simulink model "SF048A_TqLoa"  (R2013b)
settings: Solver=FixedStepDiscrete  SolverMode=SingleTasking  StartTime=0.0  StopTime=1  FixedStep=0.002  RelTol=1e-3
values from neighbouring files (symbols this model uses):
  ARCHGLBPRM_2MILLISEC_SEC_F32 = DataDict.Constant    [SF048A_TqLoa_DataDict.m]
  ARCHGLBPRM_PIOVER180_ULS_F32 = DataDict.Constant    [SF048A_TqLoa_DataDict.m]
  GRVYTLCON_MTRPERSECSQD_F32 = DataDict.Constant    [SF048A_TqLoa_DataDict.m]
  HWAUTHYMIN_ULS_F32 = DataDict.Constant    [SF048A_TqLoa_DataDict.m]
  MTRPERSECOVERKPH_MTRPERSECPERKPH_F32 = DataDict.Constant    [SF048A_TqLoa_DataDict.m]
  TqLoaDrvrTqNom = DataDict.Calibration    [SF048A_TqLoa_DataDict.m]
  TqLoaMotTqCmdLim = DataDict.Calibration    [SF048A_TqLoa_DataDict.m]
  TqLoaMotVelAndTqBasdScaFacMax = DataDict.Calibration    [SF048A_TqLoa_DataDict.m]
  TqLoaMotVelAndTqBasdScaFacMin = DataDict.Calibration    [SF048A_TqLoa_DataDict.m]
  TqLoaMotVelMgnThd = DataDict.Calibration    [SF048A_TqLoa_DataDict.m]
  TqLoaTqCmdMgnThd = DataDict.Calibration    [SF048A_TqLoa_DataDict.m]
  TqLoaVehSteerRat = DataDict.Calibration    [SF048A_TqLoa_DataDict.m]
  TqLoaVehUnderSteerGrdt = DataDict.Calibration    [SF048A_TqLoa_DataDict.m]
  TqLoaVehWhlBas = DataDict.Calibration    [SF048A_TqLoa_DataDict.m]
libraries: NxtrLim x8, FloatToFixd x5, FixdToFloat x4, LnrIntrpn x3, simulink x2, Fil x2, BilnrIntrpnCmnX x1
(part 2 of 2)

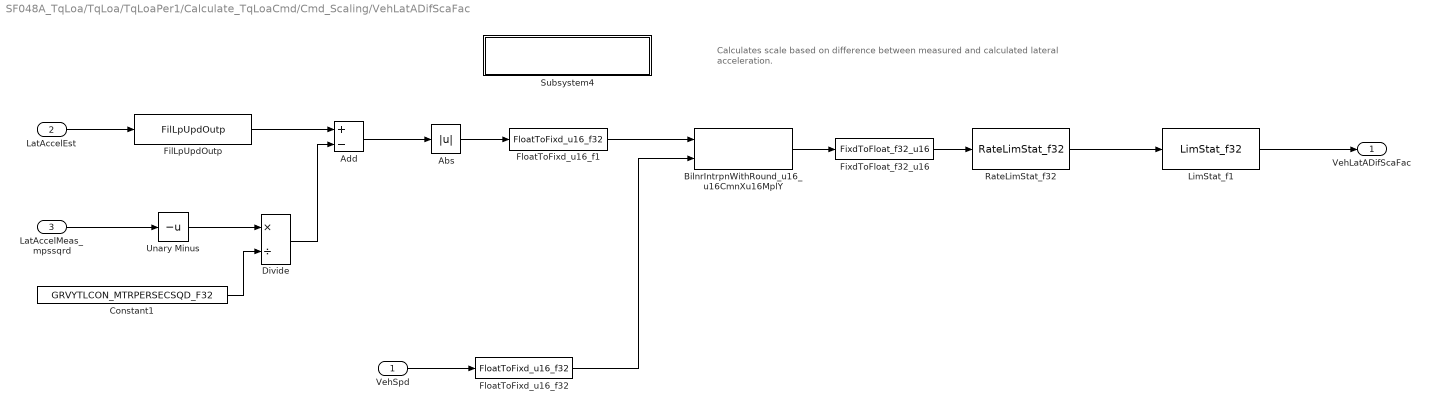
== system SF048A_TqLoa/TqLoa/TqLoaPer1/Calculate_TqLoaCmd/Cmd_Scaling/VehLatADifScaFac ==
  note: Calculates scale based on difference between measured
      | and calculated lateral acceleration.
  VehSpd : Inport
  LatAccelEst : Inport  RequirementInfo="{'linktype_rmi_doors' '0000ba57 (/E-STEER Core/SubSystem Specifications/Application Functions/SF048A Torque Sensor LOA)' '#SF048A_75' 'true' 'REQ:  SF048A_75' '' } %GIDa_e5c0702a_0213_400e_b099_5fcb4bc4666c"  Port=2
  LatAccelMeas_mpssqrd : Inport  RequirementInfo="{'linktype_rmi_doors' '0000ba57 (/E-STEER Core/SubSystem Specifications/Application Functions/SF048A Torque Sensor LOA)' '#SF048A_75' 'true' 'REQ:  SF048A_75' '' } %GIDa_d15097fd_f329_4e42_a808_1785a41628b2"  Port=3
  Abs : Abs
  Add : Sum  RequirementInfo="{'linktype_rmi_doors' '0000ba57 (/E-STEER Core/SubSystem Specifications/Application Functions/SF048A Torque Sensor LOA)' '#SF048A_75' 'true' 'REQ:  SF048A_75' '' } %GIDa_4817b60f_8b8d_4097_a7ba_bc37093a25c9"  Inputs=+-
  BilnrIntrpnWithRound_u16_u16CmnXu16MplY : BilnrIntrpnCmnX/BilnrIntrpnWithRound_u16_u16CmnXu16MplY  XTbl=TqLoaVehLatADifScaFacX  MplYTbl=TqLoaVehLatADifScaFacY  BilnrSelnTbl=TqLoaVehSpdX
      settings: AttributesFormatString=Bilnr ( u16CmnX , u16MplY )
  Constant1 : Constant  RequirementInfo="{'linktype_rmi_doors' '0000ba57 (/E-STEER Core/SubSystem Specifications/Application Functions/SF048A Torque Sensor LOA)' '#SF048A_75' 'true' 'REQ:  SF048A_75' '' } %GIDa_6e205661_965a_4c52_ae04_39f9aa3b2583"  Value=GRVYTLCON_MTRPERSECSQD_F32
  Divide : Product  RequirementInfo="{'linktype_rmi_doors' '0000ba57 (/E-STEER Core/SubSystem Specifications/Application Functions/SF048A Torque Sensor LOA)' '#SF048A_75' 'true' 'REQ:  SF048A_75' '' } %GIDa_5723e92c_a443_499a_ab6d_981db71ae68a"  Inputs=*/
  FilLpUpdOutp : Fil/FilLpUpdOutp  RequirementInfo="{'linktype_rmi_doors' '0000ba57 (/E-STEER Core/SubSystem Specifications/Application Functions/SF048A Torque Sensor LOA)' '#SF048A_75' 'true' 'REQ:  SF048A_75' '' } %GIDa_3d5f6f9b_de01_4b02_a8a7_a2d87a76a574"  StVar=VehLatAEstimnFil
      settings: AttributesFormatString=StVar: %<StVar>
  FixdToFloat_f32_u16 : FixdToFloat/FixdToFloat_f32_u16  Param1=15
  FloatToFixd_u16_f1 : FloatToFixd/FloatToFixd_u16_f32  Param1=14
  FloatToFixd_u16_f32 : FloatToFixd/FloatToFixd_u16_f32  Param1=6
  LimStat_f1 : NxtrLim/LimStat_f32  RequirementInfo="{'linktype_rmi_doors' '0000ba57 (/E-STEER Core/SubSystem Specifications/Application Functions/SF048A Torque Sensor LOA)' '#SF048A_78' 'true' 'REQ:  SF048A_78' '' } %GIDa_1186eb41_f9ab_4568_bdd1_60a08bf136a3"  LoLim=MOTTQSCAFACMIN_ULS_F32  HiLim=MOTTQSCAFACMAX_ULS_F32
      settings: AttributesFormatString=|
      | Low Limit: %<LoLim>
      | High Limit:%<HiLim>
  RateLimStat_f32 : NxtrLim/RateLimStat_f32  RequirementInfo="{'linktype_rmi_doors' '0000ba57 (/E-STEER Core/SubSystem Specifications/Application Functions/SF048A Torque Sensor LOA)' '#SF048A_77' 'true' 'REQ:  SF048A_77' '' } %GIDa_032ba997_f80f_4221_bd53_346cc12aa22e"  StVar=VehLatADifScaFacPrev  Ts=ARCHGLBPRM_2MILLISEC_SEC_F32  LoLim=TqLoaVehLatADifScaFacFallRate  HiLim=TqLoaVehLatADifScaFacRiseRate
      settings: AttributesFormatString=|
      | StVar: %<StVar>
      | LoLim: %<LoLim>
      | HiLim: %<HiLim>
  Subsystem4 : Subsystem  Description=|  mask(Copyright Information){none=on}
      | Copyright info block.                                               
      |                                                                     
      | Place copyright information at the top of every subsystem in design.
      mask prompts: none "No parameters"
      mask help: Place copyright information at the top of every subsystem in design.
      mask Display:
      | NxtrConf = 'Nexteer Confidential';
      | 
      | sys = bdroot; %handle for the current model ("system")
      | first = get_param(sys,'Created');
      | first = first(end-3:end);  %year is last four digits
      | 
      | last = get_param(sys,'LastModifiedDate');
      | if isempty(last)
      |     last = datestr(now,'yyyy');
      | else
      |     last = last(end-3:end);
      | end
      | 
      | if strcmp(first,last)
      |     fprintf('%s\nCopyright  %s Nexteer',NxtrConf,first);
      | else
      |     fprintf('%s\n%s%s-%s Nexteer',NxtrConf,char(169),first,last);
      | end
  Unary Minus : UnaryMinus  RequirementInfo="{'linktype_rmi_doors' '0000ba57 (/E-STEER Core/SubSystem Specifications/Application Functions/SF048A Torque Sensor LOA)' '#SF048A_75' 'true' 'REQ:  SF048A_75' '' } %GIDa_33a05cf1_7702_43e2_bd23_f84f74203826"
  VehLatADifScaFac : Outport
  wires:
  Divide/1 -> Add/2
  FilLpUpdOutp/1 -> Add/1
  LimStat_f1/1 -> VehLatADifScaFac/1
  LatAccelMeas_mpssqrd/1 -> Unary Minus/1
  LatAccelEst/1 -> FilLpUpdOutp/1
  Add/1 -> Abs/1
  Abs/1 -> FloatToFixd_u16_f1/1
  FloatToFixd_u16_f1/1 -> BilnrIntrpnWithRound_u16_u16CmnXu16MplY/1
  FixdToFloat_f32_u16/1 -> RateLimStat_f32/1
  RateLimStat_f32/1 -> LimStat_f1/1
  Constant1/1 -> Divide/2
  Unary Minus/1 -> Divide/1
  VehSpd/1 -> FloatToFixd_u16_f32/1
  BilnrIntrpnWithRound_u16_u16CmnXu16MplY/1 -> FixdToFloat_f32_u16/1
  FloatToFixd_u16_f32/1 -> BilnrIntrpnWithRound_u16_u16CmnXu16MplY/2

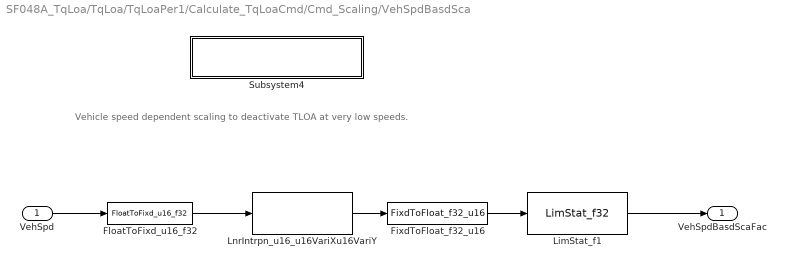
== system SF048A_TqLoa/TqLoa/TqLoaPer1/Calculate_TqLoaCmd/Cmd_Scaling/VehSpdBasdSca ==
  note: Vehicle speed dependent scaling to deactivate TLOA at very low speeds.
  VehSpd : Inport  RequirementInfo="{'linktype_rmi_doors' '0000ba57 (/E-STEER Core/SubSystem Specifications/Application Functions/SF048A Torque Sensor LOA)' '#SF048A_71' 'true' 'REQ:  SF048A_71' '' } %GIDa_e22fb202_c1ea_42b7_b8f3_811ad6335ef5"
  FixdToFloat_f32_u16 : FixdToFloat/FixdToFloat_f32_u16  Param1=15
  FloatToFixd_u16_f32 : FloatToFixd/FloatToFixd_u16_f32  RequirementInfo="{'linktype_rmi_doors' '0000ba57 (/E-STEER Core/SubSystem Specifications/Application Functions/SF048A Torque Sensor LOA)' '#SF048A_71' 'true' 'REQ:  SF048A_71' '' } %GIDa_f395791a_d0c7_43ab_b916_b2cb557517b6"  Param1=6
  LimStat_f1 : NxtrLim/LimStat_f32  RequirementInfo="{'linktype_rmi_doors' '0000ba57 (/E-STEER Core/SubSystem Specifications/Application Functions/SF048A Torque Sensor LOA)' '#SF048A_72' 'true' 'REQ:  SF048A_72' '' } %GIDa_8703505f_376b_4477_881a_364f92790bea"  LoLim=MOTTQSCAFACMIN_ULS_F32  HiLim=MOTTQSCAFACMAX_ULS_F32
      settings: AttributesFormatString=|
      | Low Limit: %<LoLim>
      | High Limit:%<HiLim>
  LnrIntrpn_u16_u16VariXu16VariY : LnrIntrpn/LnrIntrpn_u16_u16VariXu16VariY  RequirementInfo="{'linktype_rmi_doors' '0000ba57 (/E-STEER Core/SubSystem Specifications/Application Functions/SF048A Torque Sensor LOA)' '#SF048A_71' 'true' 'REQ:  SF048A_71' '' } %GIDa_3086bf50_8e4c_4a7b_9825_1eb9b0ca8a87"  XTbl=TqLoaVehSpdScaFacX  YTbl=TqLoaVehSpdScaFacY
      settings: AttributesFormatString=Lnr ( u16VariX , u16VariY )
  Subsystem4 : Subsystem  Description=|  mask(Copyright Information){none=on}
      | Copyright info block.                                               
      |                                                                     
      | Place copyright information at the top of every subsystem in design.
      mask prompts: none "No parameters"
      mask help: Place copyright information at the top of every subsystem in design.
      mask Display:
      | NxtrConf = 'Nexteer Confidential';
      | 
      | sys = bdroot; %handle for the current model ("system")
      | first = get_param(sys,'Created');
      | first = first(end-3:end);  %year is last four digits
      | 
      | last = get_param(sys,'LastModifiedDate');
      | if isempty(last)
      |     last = datestr(now,'yyyy');
      | else
      |     last = last(end-3:end);
      | end
      | 
      | if strcmp(first,last)
      |     fprintf('%s\nCopyright  %s Nexteer',NxtrConf,first);
      | else
      |     fprintf('%s\n%s%s-%s Nexteer',NxtrConf,char(169),first,last);
      | end
  VehSpdBasdScaFac : Outport
  wires:
  LnrIntrpn_u16_u16VariXu16VariY/1 -> FixdToFloat_f32_u16/1
  VehSpd/1 -> FloatToFixd_u16_f32/1
  FixdToFloat_f32_u16/1 -> LimStat_f1/1
  FloatToFixd_u16_f32/1 -> LnrIntrpn_u16_u16VariXu16VariY/1
  LimStat_f1/1 -> VehSpdBasdScaFac/1

== system SF048A_TqLoa/TqLoa/TqLoaPer1/ValidityCheck/If Action Subsystem/Subsystem4 ==

== system SF048A_TqLoa/TqLoa/TqLoaPer1/ValidityCheck/If Action Subsystem1/Subsystem4 ==

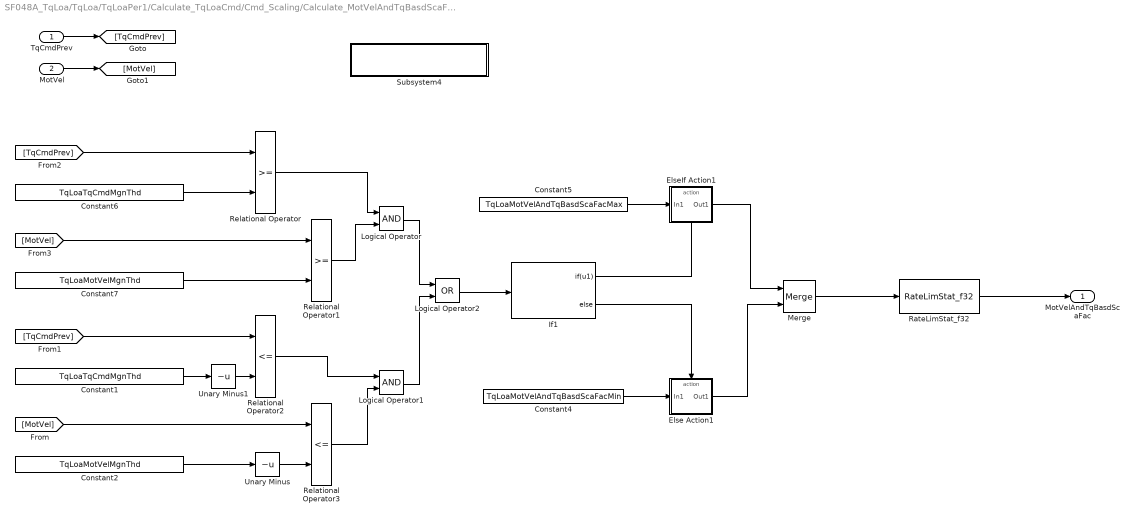
== system SF048A_TqLoa/TqLoa/TqLoaPer1/Calculate_TqLoaCmd/Cmd_Scaling/Calculate_MotVelAndTqBasdScaFac/Calculate MotVelAndTqBasdScaFac ==
  TqCmdPrev : Inport
  MotVel : Inport  Port=2
  Constant1 : Constant  RequirementInfo="{'linktype_rmi_doors' '0000ba57 (/E-STEER Core/SubSystem Specifications/Application Functions/SF048A Torque Sensor LOA)' '#SF048A_66' 'true' 'REQ:  SF048A_66' '' ; 'linktype_rmi_doors' '0000ba57 (/E-STEER Core/SubSystem Specifications/Application Functions/SF048A Torque Sensor LOA)' '#SF048A_67' 'true' 'REQ:  SF048A_67' '' } %GIDa_bdc127ed_d37b_41c9_97be_c7ba18402397"  Value=TqLoaTqCmdMgnThd
  Constant2 : Constant  RequirementInfo="{'linktype_rmi_doors' '0000ba57 (/E-STEER Core/SubSystem Specifications/Application Functions/SF048A Torque Sensor LOA)' '#SF048A_66' 'true' 'REQ:  SF048A_66' '' ; 'linktype_rmi_doors' '0000ba57 (/E-STEER Core/SubSystem Specifications/Application Functions/SF048A Torque Sensor LOA)' '#SF048A_67' 'true' 'REQ:  SF048A_67' '' } %GIDa_dacd5d55_a79f_4acb_a8a4_d1ab007f0fa6"  Value=TqLoaMotVelMgnThd
  Constant4 : Constant  RequirementInfo="{'linktype_rmi_doors' '0000ba57 (/E-STEER Core/SubSystem Specifications/Application Functions/SF048A Torque Sensor LOA)' '#SF048A_67' 'true' 'REQ:  SF048A_67' '' } %GIDa_c59c1821_1927_4d51_8dc4_9290abcf5d28"  Value=TqLoaMotVelAndTqBasdScaFacMin  OutDataTypeStr=single
  Constant5 : Constant  RequirementInfo="{'linktype_rmi_doors' '0000ba57 (/E-STEER Core/SubSystem Specifications/Application Functions/SF048A Torque Sensor LOA)' '#SF048A_66' 'true' 'REQ:  SF048A_66' '' } %GIDa_8b5dc1f4_6803_4763_ac92_0d4a41fb14a6"  Value=TqLoaMotVelAndTqBasdScaFacMax  OutDataTypeStr=single
  Constant6 : Constant  RequirementInfo="{'linktype_rmi_doors' '0000ba57 (/E-STEER Core/SubSystem Specifications/Application Functions/SF048A Torque Sensor LOA)' '#SF048A_66' 'true' 'REQ:  SF048A_66' '' ; 'linktype_rmi_doors' '0000ba57 (/E-STEER Core/SubSystem Specifications/Application Functions/SF048A Torque Sensor LOA)' '#SF048A_67' 'true' 'REQ:  SF048A_67' '' } %GIDa_00a9b28c_8bba_4162_8ef2_448d44ca4708"  Value=TqLoaTqCmdMgnThd
  Constant7 : Constant  RequirementInfo="{'linktype_rmi_doors' '0000ba57 (/E-STEER Core/SubSystem Specifications/Application Functions/SF048A Torque Sensor LOA)' '#SF048A_66' 'true' 'REQ:  SF048A_66' '' ; 'linktype_rmi_doors' '0000ba57 (/E-STEER Core/SubSystem Specifications/Application Functions/SF048A Torque Sensor LOA)' '#SF048A_67' 'true' 'REQ:  SF048A_67' '' } %GIDa_a7bc639d_cde0_4a2d_a632_5bcfa70e1b2b"  Value=TqLoaMotVelMgnThd
  Else Action1 : Subsystem  RequirementInfo="{'linktype_rmi_doors' '0000ba57 (/E-STEER Core/SubSystem Specifications/Application Functions/SF048A Torque Sensor LOA)' '#SF048A_67' 'true' 'REQ:  SF048A_67' '' } %GIDa_55e6e90c_135f_4880_9e1b_2480b15c4e52"  TreatAsAtomicUnit=on
  ElseIf Action1 : Subsystem  RequirementInfo="{'linktype_rmi_doors' '0000ba57 (/E-STEER Core/SubSystem Specifications/Application Functions/SF048A Torque Sensor LOA)' '#SF048A_66' 'true' 'REQ:  SF048A_66' '' } %GIDa_94bea9dd_8a09_46dd_afe4_dfca7bf7cfd1"  TreatAsAtomicUnit=on
  If1 : If  RequirementInfo="{'linktype_rmi_doors' '0000ba57 (/E-STEER Core/SubSystem Specifications/Application Functions/SF048A Torque Sensor LOA)' '#SF048A_66' 'true' 'REQ:  SF048A_66' '' ; 'linktype_rmi_doors' '0000ba57 (/E-STEER Core/SubSystem Specifications/Application Functions/SF048A Torque Sensor LOA)' '#SF048A_67' 'true' 'REQ:  SF048A_67' '' } %GIDa_026e03a9_9b19_414d_9f25_a0fdee78621e"  IfExpression=u1
  Logical Operator : Logic  RequirementInfo="{'linktype_rmi_doors' '0000ba57 (/E-STEER Core/SubSystem Specifications/Application Functions/SF048A Torque Sensor LOA)' '#SF048A_66' 'true' 'REQ:  SF048A_66' '' ; 'linktype_rmi_doors' '0000ba57 (/E-STEER Core/SubSystem Specifications/Application Functions/SF048A Torque Sensor LOA)' '#SF048A_67' 'true' 'REQ:  SF048A_67' '' } %GIDa_3065d4cf_6eff_4026_bf75_931b6f2c20a1"  AllPortsSameDT=off  OutDataTypeStr=boolean
  Logical Operator1 : Logic  RequirementInfo="{'linktype_rmi_doors' '0000ba57 (/E-STEER Core/SubSystem Specifications/Application Functions/SF048A Torque Sensor LOA)' '#SF048A_66' 'true' 'REQ:  SF048A_66' '' ; 'linktype_rmi_doors' '0000ba57 (/E-STEER Core/SubSystem Specifications/Application Functions/SF048A Torque Sensor LOA)' '#SF048A_67' 'true' 'REQ:  SF048A_67' '' } %GIDa_fcef087c_dc44_410f_a5a0_1ffe5fff2f34"  AllPortsSameDT=off  OutDataTypeStr=boolean
  Logical Operator2 : Logic  RequirementInfo="{'linktype_rmi_doors' '0000ba57 (/E-STEER Core/SubSystem Specifications/Application Functions/SF048A Torque Sensor LOA)' '#SF048A_66' 'true' 'REQ:  SF048A_66' '' ; 'linktype_rmi_doors' '0000ba57 (/E-STEER Core/SubSystem Specifications/Application Functions/SF048A Torque Sensor LOA)' '#SF048A_67' 'true' 'REQ:  SF048A_67' '' } %GIDa_e796ba44_6874_451e_b9aa_cf4f7b691495"  Operator=OR  AllPortsSameDT=off  OutDataTypeStr=boolean
  Merge : Merge
  RateLimStat_f32 : NxtrLim/RateLimStat_f32  RequirementInfo="{'linktype_rmi_doors' '0000ba57 (/E-STEER Core/SubSystem Specifications/Application Functions/SF048A Torque Sensor LOA)' '#SF048A_68' 'true' 'REQ:  SF048A_68' '' } %GIDa_a92a6012_f14b_4094_87df_c479bd942f9c"  StVar=MotVelAndTqBasdScaFacPrev  Ts=ARCHGLBPRM_2MILLISEC_SEC_F32  LoLim=TqLoaMotVelAndTqBasdScaFacFallRate  HiLim=TqLoaMotVelAndTqBasdScaFacRiseRate
      settings: AttributesFormatString=|
      | StVar: %<StVar>
      | LoLim: %<LoLim>
      | HiLim: %<HiLim>
  Relational Operator : RelationalOperator  RequirementInfo="{'linktype_rmi_doors' '0000ba57 (/E-STEER Core/SubSystem Specifications/Application Functions/SF048A Torque Sensor LOA)' '#SF048A_66' 'true' 'REQ:  SF048A_66' '' ; 'linktype_rmi_doors' '0000ba57 (/E-STEER Core/SubSystem Specifications/Application Functions/SF048A Torque Sensor LOA)' '#SF048A_67' 'true' 'REQ:  SF048A_67' '' } %GIDa_5857ce7c_9f74_46ef_83b4_df296295cbeb"  OutDataTypeStr=boolean
  Relational Operator1 : RelationalOperator  RequirementInfo="{'linktype_rmi_doors' '0000ba57 (/E-STEER Core/SubSystem Specifications/Application Functions/SF048A Torque Sensor LOA)' '#SF048A_66' 'true' 'REQ:  SF048A_66' '' ; 'linktype_rmi_doors' '0000ba57 (/E-STEER Core/SubSystem Specifications/Application Functions/SF048A Torque Sensor LOA)' '#SF048A_67' 'true' 'REQ:  SF048A_67' '' } %GIDa_9a0f7820_223f_42af_a006_23917ce02771"  OutDataTypeStr=boolean
  Relational Operator2 : RelationalOperator  RequirementInfo="{'linktype_rmi_doors' '0000ba57 (/E-STEER Core/SubSystem Specifications/Application Functions/SF048A Torque Sensor LOA)' '#SF048A_66' 'true' 'REQ:  SF048A_66' '' ; 'linktype_rmi_doors' '0000ba57 (/E-STEER Core/SubSystem Specifications/Application Functions/SF048A Torque Sensor LOA)' '#SF048A_67' 'true' 'REQ:  SF048A_67' '' } %GIDa_5ee6ae7f_bdbd_4808_bfb0_6fe7c170d98f"  Operator=<=  OutDataTypeStr=boolean
  Relational Operator3 : RelationalOperator  RequirementInfo="{'linktype_rmi_doors' '0000ba57 (/E-STEER Core/SubSystem Specifications/Application Functions/SF048A Torque Sensor LOA)' '#SF048A_66' 'true' 'REQ:  SF048A_66' '' ; 'linktype_rmi_doors' '0000ba57 (/E-STEER Core/SubSystem Specifications/Application Functions/SF048A Torque Sensor LOA)' '#SF048A_67' 'true' 'REQ:  SF048A_67' '' } %GIDa_195e5406_f3bd_4d81_a3cb_ec970f7cd8b3"  Operator=<=  OutDataTypeStr=boolean
  Subsystem4 : Subsystem  Description=|  mask(Copyright Information){none=on}
      | Copyright info block.                                               
      |                                                                     
      | Place copyright information at the top of every subsystem in design.
      mask prompts: none "No parameters"
      mask help: Place copyright information at the top of every subsystem in design.
      mask Display:
      | NxtrConf = 'Nexteer Confidential';
      | 
      | sys = bdroot; %handle for the current model ("system")
      | first = get_param(sys,'Created');
      | first = first(end-3:end);  %year is last four digits
      | 
      | last = get_param(sys,'LastModifiedDate');
      | if isempty(last)
      |     last = datestr(now,'yyyy');
      | else
      |     last = last(end-3:end);
      | end
      | 
      | if strcmp(first,last)
      |     fprintf('%s\nCopyright  %s Nexteer',NxtrConf,first);
      | else
      |     fprintf('%s\n%s%s-%s Nexteer',NxtrConf,char(169),first,last);
      | end
  Unary Minus : UnaryMinus  RequirementInfo="{'linktype_rmi_doors' '0000ba57 (/E-STEER Core/SubSystem Specifications/Application Functions/SF048A Torque Sensor LOA)' '#SF048A_66' 'true' 'REQ:  SF048A_66' '' ; 'linktype_rmi_doors' '0000ba57 (/E-STEER Core/SubSystem Specifications/Application Functions/SF048A Torque Sensor LOA)' '#SF048A_67' 'true' 'REQ:  SF048A_67' '' } %GIDa_9c369332_5f2c_44c1_b114_efd3576bd965"
  Unary Minus1 : UnaryMinus  RequirementInfo="{'linktype_rmi_doors' '0000ba57 (/E-STEER Core/SubSystem Specifications/Application Functions/SF048A Torque Sensor LOA)' '#SF048A_66' 'true' 'REQ:  SF048A_66' '' ; 'linktype_rmi_doors' '0000ba57 (/E-STEER Core/SubSystem Specifications/Application Functions/SF048A Torque Sensor LOA)' '#SF048A_67' 'true' 'REQ:  SF048A_67' '' } %GIDa_1b8a2ab4_12fe_4aa9_868c_b9ad48dde733"
  MotVelAndTqBasdScaFac : Outport
  wires:
  Constant6/1 -> Relational Operator/2
  Relational Operator/1 -> Logical Operator/1
  Constant7/1 -> Relational Operator1/2
  Relational Operator1/1 -> Logical Operator/2
  Else Action1/1(Out1) -> Merge/2
  Constant4/1 -> Else Action1/1(In1)
  If1/2 -> Else Action1/Action
  Constant5/1 -> ElseIf Action1/1(In1)
  If1/1 -> ElseIf Action1/Action
  ElseIf Action1/1(Out1) -> Merge/1
  Merge/1 -> RateLimStat_f32/1
  RateLimStat_f32/1 -> MotVelAndTqBasdScaFac/1
  Constant1/1 -> Unary Minus1/1
  Relational Operator2/1 -> Logical Operator1/1
  Constant2/1 -> Unary Minus/1
  Relational Operator3/1 -> Logical Operator1/2
  Unary Minus/1 -> Relational Operator3/2
  Unary Minus1/1 -> Relational Operator2/2
  Logical Operator1/1 -> Logical Operator2/2
  Logical Operator/1 -> Logical Operator2/1
  Logical Operator2/1 -> If1/1
  TqCmdPrev/1 -> [TqCmdPrev]
  MotVel/1 -> [MotVel]
  [MotVel] -> Relational Operator3/1
  [TqCmdPrev] -> Relational Operator2/1
  [MotVel] -> Relational Operator1/1
  [TqCmdPrev] -> Relational Operator/1

== system SF048A_TqLoa/TqLoa/TqLoaPer1/Calculate_TqLoaCmd/Cmd_Scaling/Calculate_MotVelAndTqBasdScaFac/Subsystem4 ==

== system SF048A_TqLoa/TqLoa/TqLoaPer1/Calculate_TqLoaCmd/Cmd_Scaling/VehLatADifScaFac/Subsystem4 ==

== system SF048A_TqLoa/TqLoa/TqLoaPer1/Calculate_TqLoaCmd/Cmd_Scaling/VehSpdBasdSca/Subsystem4 ==

== system SF048A_TqLoa/TqLoa/TqLoaPer1/Calculate_TqLoaCmd/Cmd_Scaling/Calculate_MotVelAndTqBasdScaFac/Calculate MotVelAndTqBasdScaFac/Else Action1 ==
  In1 : Inport
  Action Port : ActionPort  ActionType=else
  Subsystem4 : Subsystem  Description=|  mask(Copyright Information){none=on}
      | Copyright info block.                                               
      |                                                                     
      | Place copyright information at the top of every subsystem in design.
      mask prompts: none "No parameters"
      mask help: Place copyright information at the top of every subsystem in design.
      mask Display:
      | NxtrConf = 'Nexteer Confidential';
      | 
      | sys = bdroot; %handle for the current model ("system")
      | first = get_param(sys,'Created');
      | first = first(end-3:end);  %year is last four digits
      | 
      | last = get_param(sys,'LastModifiedDate');
      | if isempty(last)
      |     last = datestr(now,'yyyy');
      | else
      |     last = last(end-3:end);
      | end
      | 
      | if strcmp(first,last)
      |     fprintf('%s\nCopyright  %s Nexteer',NxtrConf,first);
      | else
      |     fprintf('%s\n%s%s-%s Nexteer',NxtrConf,char(169),first,last);
      | end
  Out1 : Outport
  wires:
  In1/1 -> Out1/1

== system SF048A_TqLoa/TqLoa/TqLoaPer1/Calculate_TqLoaCmd/Cmd_Scaling/Calculate_MotVelAndTqBasdScaFac/Calculate MotVelAndTqBasdScaFac/ElseIf Action1 ==
  In1 : Inport
  Action Port : ActionPort  ActionType=then
  Subsystem4 : Subsystem  Description=|  mask(Copyright Information){none=on}
      | Copyright info block.                                               
      |                                                                     
      | Place copyright information at the top of every subsystem in design.
      mask prompts: none "No parameters"
      mask help: Place copyright information at the top of every subsystem in design.
      mask Display:
      | NxtrConf = 'Nexteer Confidential';
      | 
      | sys = bdroot; %handle for the current model ("system")
      | first = get_param(sys,'Created');
      | first = first(end-3:end);  %year is last four digits
      | 
      | last = get_param(sys,'LastModifiedDate');
      | if isempty(last)
      |     last = datestr(now,'yyyy');
      | else
      |     last = last(end-3:end);
      | end
      | 
      | if strcmp(first,last)
      |     fprintf('%s\nCopyright  %s Nexteer',NxtrConf,first);
      | else
      |     fprintf('%s\n%s%s-%s Nexteer',NxtrConf,char(169),first,last);
      | end
  Out1 : Outport
  wires:
  In1/1 -> Out1/1

== system SF048A_TqLoa/TqLoa/TqLoaPer1/Calculate_TqLoaCmd/Cmd_Scaling/Calculate_MotVelAndTqBasdScaFac/Calculate MotVelAndTqBasdScaFac/Subsystem4 ==

== system SF048A_TqLoa/TqLoa/TqLoaPer1/Calculate_TqLoaCmd/Cmd_Scaling/Calculate_MotVelAndTqBasdScaFac/Calculate MotVelAndTqBasdScaFac/Else Action1/Subsystem4 ==

== system SF048A_TqLoa/TqLoa/TqLoaPer1/Calculate_TqLoaCmd/Cmd_Scaling/Calculate_MotVelAndTqBasdScaFac/Calculate MotVelAndTqBasdScaFac/ElseIf Action1/Subsystem4 ==
